simulink model "absolute"  (R2017a)
settings: Solver=VariableStepAuto  StartTime=0.0  StopTime=10.0  RelTol=1e-3
undefined symbols (not defined in the file): contractAfterSimulation, contractBeforeSimulation, ContractBlock, ContractGuaranteeBlock, ContractValidatorBlock, saveValidatorParameters
libraries: simulink x2
settings Model: Creator=mahgoubyahia  LastModifiedBy=mahgoubyahia

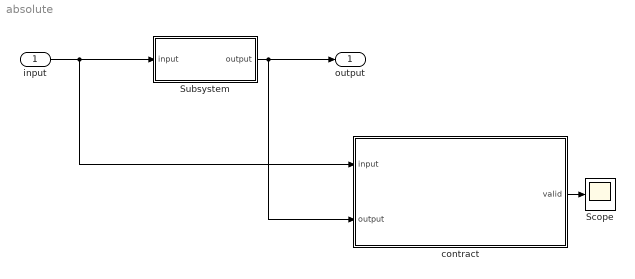
== system absolute ==
  input : Inport  OutDataTypeStr=int32
  Scope : Scope
  Subsystem : Subsystem
  contract : Subsystem  mask{ContractBlockType=ContractBlock}
      mask init:
      | set_param(gcb, 'LinkStatus', 'none');
      mask DialogControl DescTextVar Prompt: Contract block
      mask Display:
      | text(0.5, 0.5, '{\bf\fontsize{20}Contract}', 'hor', 'center', 'texmode','on');
      | blocks = find_system(gcb, 'LookUnderMasks','all', 'SearchDepth',1,'BlockType','Inport');
      | for i = 1 : length(blocks)
      |     blockName = get_param(blocks(i), 'Name');
      |     [path, blockName] = fileparts(char(blockName));
      |     port_label('input', i, blockName);
      | end
      | 
      | blocks = find_system(gcb, 'LookUnderMasks','all', 'SearchDepth',1,'BlockType','Outport');
      | for i = 1 : length(blocks)
      |     blockName = get_param(blocks(i), 'Name');
      |     [path, blockName] = fileparts(char(blockName));
      |     port_label('output', i, blockName);
      | end
  output : Outport
  wires:
  input/1 -> contract/1(input), Subsystem/1(input)
  contract/1(valid) -> Scope/1
  Subsystem/1(output) -> contract/2(output), output/1

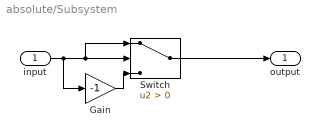
== system absolute/Subsystem ==
  input : Inport
  Gain : Gain  Gain=-1  OutDataTypeStr=int32
  Switch : Switch  Criteria=u2 > Threshold
  output : Outport
  wires:
  Switch/1 -> output/1
  input/1 -> Gain/1, Switch/1, Switch/2
  Gain/1 -> Switch/3

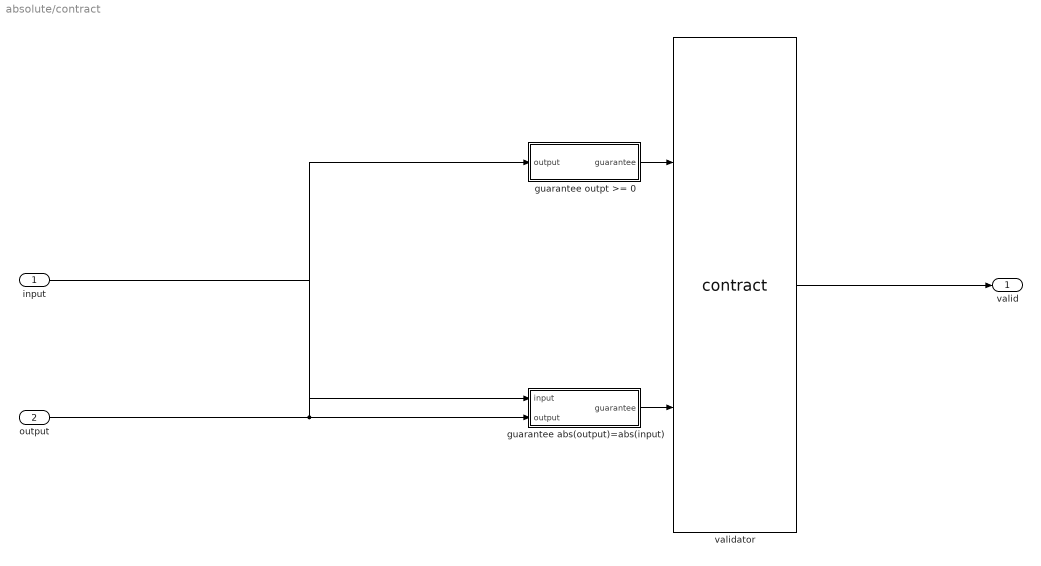
== system absolute/contract ==
  input : Inport  OutDataTypeStr=int32
  output : Inport  Port=2  OutDataTypeStr=int32
  guarantee abs(output)=abs(input) : Subsystem  mask{ContractBlockType=ContractGuaranteeBlock}
      mask init:
      | set_param(gcb, 'LinkStatus', 'none');
      mask DialogControl DescTextVar Prompt: Guarantee block
  guarantee outpt >= 0 : Subsystem  mask{ContractBlockType=ContractGuaranteeBlock}
      mask init:
      | set_param(gcb, 'LinkStatus', 'none');
      mask DialogControl DescTextVar Prompt: Guarantee block
  validator : M-S-Function  LoadFcn=saveValidatorParameters(gcb);  InitFcn=contractBeforeSimulation();  StopFcn=contractAfterSimulation();  FunctionName=contract  mask{assumePorts=0, guaranteePorts=2, modePorts=0, ContractBlockType=ContractValidatorBlock, createInportsCheckbox=on, createEnsureRequireCheckbox=on}
      mask prompts: assumePorts "Assume ports     :"; guaranteePorts "Guarantee ports :"; modePorts "Mode ports        :"; createInportsCheckbox "Create inports and connect them automatically"; createEnsureRequireCheckbox "Create ensure and require blocks for mode blocks"
      mask init:
      | set_param(gcb,'LinkStatus','none');
      | contract_callback('inputs_callback',gcb);
      mask DialogControl DescTextVar Prompt: The validator block implements the following logic: <br> <br> <b>Sofar</b>(assume<sub>1</sub> <b>&#8743;</b> assume<sub>2</sub> <b>&#8743;</b> ... assume<sub>k</sub>) <b>&rarr;</b> (guarantee<sub>1</sub> <b>&#8743;</b> guarantee<sub>2</sub> <b>&#8743;</b> ... guarantee<sub>m</sub> <b>&#8743;</b>  mode<sub>1</sub> <b>&#8743;</b> mode<sub>2</sub> <b>&#8743;</b> ... <b>&#8743;</b> mode<sub>n</sub> )<br> where mode<sub>i</sub> = require<sub>i</sub> <b>&rarr;</b> ensure<sub>i</sub>
      mask Display:
      | port_label('input',1,'guarantee')
      | port_label('input',2,'guarantee')
      | port_label('output',1,'valid')
  valid : Outport
  wires:
  validator/1 -> valid/1
  input/1 -> guarantee abs(output)=abs(input)/1(input)
  output/1 -> guarantee abs(output)=abs(input)/2(output), guarantee outpt >= 0/1(output)
  guarantee abs(output)=abs(input)/1(guarantee) -> validator/2
  guarantee outpt >= 0/1(guarantee) -> validator/1

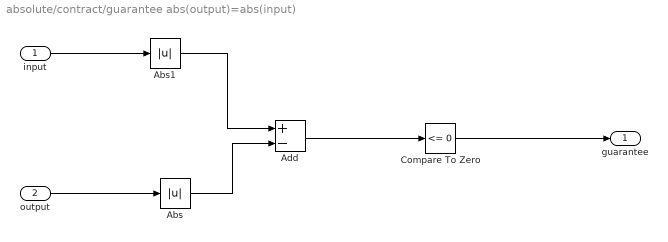
== system absolute/contract/guarantee abs(output)=abs(input) ==
  input : Inport
  output : Inport  Port=2
  Abs : Abs
  Abs1 : Abs
  Add : Sum  Inputs=+-
  Compare To Zero : simulink/Logic and Bit Operations/Compare To Zero  relop=<=  OutDataTypeStr=boolean
  guarantee : Outport  OutDataTypeStr=boolean
  wires:
  output/1 -> Abs/1
  input/1 -> Abs1/1
  Abs1/1 -> Add/1
  Abs/1 -> Add/2
  Add/1 -> Compare To Zero/1
  Compare To Zero/1 -> guarantee/1

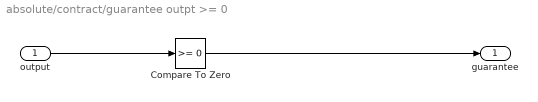
== system absolute/contract/guarantee outpt >= 0 ==
  output : Inport
  Compare To Zero : simulink/Logic and Bit Operations/Compare To Zero  relop=>=  OutDataTypeStr=boolean
  guarantee : Outport  OutDataTypeStr=boolean
  wires:
  output/1 -> Compare To Zero/1
  Compare To Zero/1 -> guarantee/1
